simulink model "one_dof_free_oscillations"  (R2019a)
settings: Solver=VariableStepAuto  StartTime=0.0  StopTime=time_span(end)  RelTol=1e-3
values from neighbouring files (symbols this model uses):
  c = 0    [one_dof_solver_symbolically.m]    (also in one_dof_system_free_oscillations.m; onedof_system_numerical_solution.m = 1000)
  k = 50000    [one_dof_solver_symbolically.m]    (also in one_dof_system_free_oscillations.m; onedof_system_numerical_solution.m)
  m = 750    [one_dof_solver_symbolically.m]    (also in one_dof_system_free_oscillations.m; onedof_system_numerical_solution.m)
  x_0 = 0.01    [one_dof_solver_symbolically.m]    (also in one_dof_system_free_oscillations.m; onedof_system_numerical_solution.m)
  xdot_0 = 0    [one_dof_system_free_oscillations.m]    (also in onedof_system_numerical_solution.m)
settings Model: Creator=HP  LastModifiedBy=HP

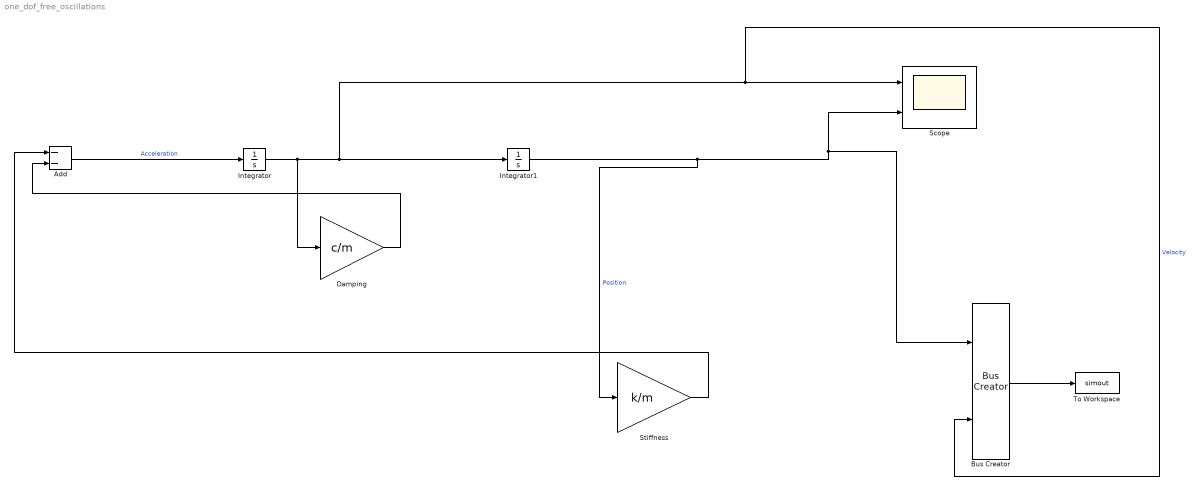
== system one_dof_free_oscillations ==
  Add : Sum  Inputs=--
  Bus Creator : BusCreator  Inputs=2
  "Damping " : Gain  Gain=c/m
  Integrator : Integrator  InitialCondition=xdot_0
  Integrator1 : Integrator  InitialCondition=x_0
  Scope : Scope  NumInputPorts=2
  Stiffness : Gain  Gain=k/m
  To Workspace : ToWorkspace  VariableName=simout  SaveFormat=Timeseries  SampleTime=-1
  wires:
  Integrator/1 -> "Damping "/1, Bus Creator/2, Scope/1, Integrator1/1  "Velocity"
  Integrator1/1 -> Scope/2, Bus Creator/1, Stiffness/1  "Position"
  Bus Creator/1 -> To Workspace/1
  "Damping "/1 -> Add/2
  Stiffness/1 -> Add/1
  Add/1 -> Integrator/1  "Acceleration"
